simulink model "LinearIntegralAntiWindup"  (R2024b)
settings: Solver=FixedStepAuto  StartTime=0  StopTime=120  FixedStep=0.002  RelTol=1e-3
model workspace (MAT data in the model file):
  Disturbance : Simulink.Parameter (value not decoded)
  ToDrvDesigner : Simulink.Parameter (value not decoded)
values from neighbouring files (symbols this model uses):
  C_af = 80000.0    [VehicleData.sldd]
  C_ar = 80000.0    [VehicleData.sldd]
  g = 9.81    [VehicleData.sldd]
  Iz = 2873.0    [VehicleData.sldd]
  lf = 1.1    [VehicleData.sldd]
  lr = 1.58    [VehicleData.sldd]
  m = 2238.932    [VehicleData.sldd]
symbols that are objects in the model workspace (value not decoded): Disturbance
undefined symbols (not defined in the file or in its folder): phi
libraries: slpidlib x9, SignalEditorBlockLib x1
(part 2 of 3)

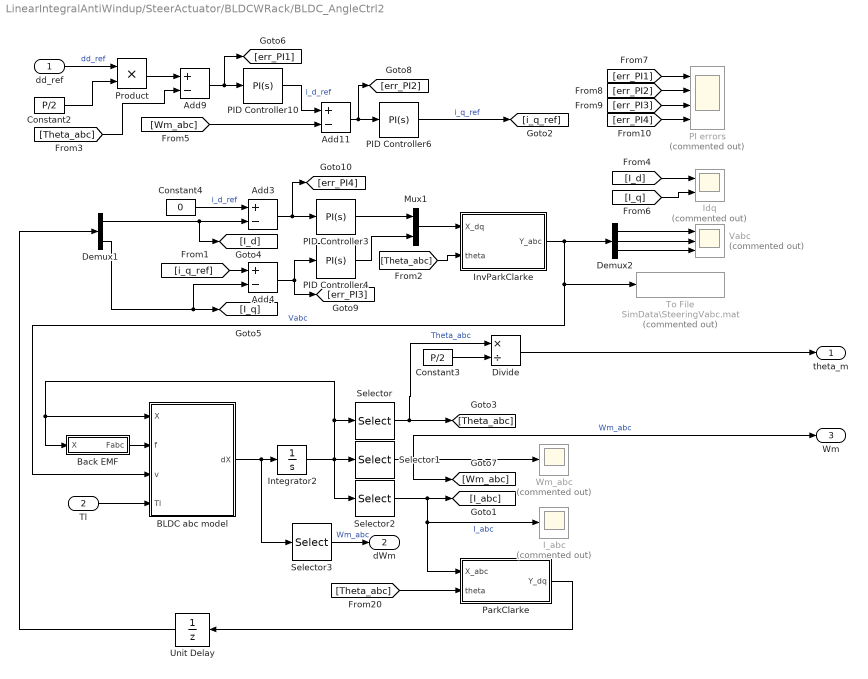
== system LinearIntegralAntiWindup/SteerActuator/BLDCWRack/BLDC_AngleCtrl2 ==
  dd_ref : Inport
  Tl : Inport  Port=2
  Add{3..4,9,11} (4 alike) : Sum  Inputs=+-
  BLDC abc model : MATLAB Function  TreatAsAtomicUnit=on
  Back EMF : MATLAB Function  TreatAsAtomicUnit=on
  Constant2 : Constant  Value=P/2
  Constant3 : Constant  Value=P/2
  Constant4 : Constant  Value=0
  Demux1 : Demux  Outputs=2
  Demux2 : Demux  Outputs=3
  Divide : Product  Inputs=*/
  I_abc : Scope  Commented=on
  Idq : Scope  Commented=on  NumInputPorts=2
  Integrator2 : Integrator  InitialCondition=[0;0;0;0.1;0]
  InvParkClarke : MATLAB Function  TreatAsAtomicUnit=on
  Mux1 : Mux  Inputs=2
  PI errors : Scope  Commented=on  NumInputPorts=4
  PID Controller10 : slpidlib/PID Controller  Controller=PI  Form=Parallel  TimeDomain=Continuous-time  UseExternalTs=off  SampleTime=-1  IntegratorMethod=Forward Euler  FilterMethod=Forward Euler  ControllerParametersSource=internal  P=50  I=2  UseKiTs=off  D=0  UseExternalDerivativeSource=off  N=100  UseFilter=on  TunerSelectOption=Transfer Function Based (PID Tuner App)  InitialConditionSource=internal  InitialConditionForIntegrator=0  InitialConditionForFilter=0  DifferentiatorICPrevScaledInput=0  ExternalReset=none  TrackingMode=off  Kt=1  LimitOutput=off  SatLimitsSource=internal  UpperSaturationLimit=500  LowerSaturationLimit=-500  LinearizeAsGain=on  AntiWindupMode=back-calculation  Kb=1  LimitIntegrator=off  UpperIntegratorSaturationLimit=inf  LowerIntegratorSaturationLimit=-inf  POutMin=[]  POutMax=[]  IOutMin=[]  IOutMax=[]  DOutMin=[]  DOutMax=[]  NOutMin=[]  NOutMax=[]  SumOutMin=[]  SumOutMax=[]  SaturationOutMin=[]  SaturationOutMax=[]  PParamMin=[]  PParamMax=[]  IParamMin=[]  IParamMax=[]  DParamMin=[]  DParamMax=[]  NParamMin=[]  NParamMax=[]  KbParamMin=[]  KbParamMax=[]  KtParamMin=[]  KtParamMax=[]  KbOutMin=[]  KbOutMax=[]  KtOutMin=[]  KtOutMax=[]  IntegratorOutMin=[]  IntegratorOutMax=[]  FilterOutMin=[]  FilterOutMax=[]  SumI1OutMin=[]  SumI1OutMax=[]  SumI2OutMin=[]  SumI2OutMax=[]  SumI3OutMin=[]  SumI3OutMax=[]  SumI4OutMin=[]  SumI4OutMax=[]  SumDOutMin=[]  SumDOutMax=[]  DifferentiatorOutMin=[]  DifferentiatorOutMax=[]  FilterDiffOutCoefMin=[]  FilterDiffOutCoefMax=[]  ReciprocalOutMin=[]  ReciprocalOutMax=[]  SumDenOutMin=[]  SumDenOutMax=[]  SumNumOutMin=[]  SumNumOutMax=[]  DivideOutMin=[]  DivideOutMax=[]  UdiffTsProdOutMin=[]  UdiffTsProdOutMax=[]  NTsProdOutMin=[]  NTsProdOutMax=[]  UintegralTsProdOutMin=[]  UintegralTsProdOutMax=[]  UngainTsProdOutMin=[]  UngainTsProdOutMax=[]  ClampingZeroOutDataTypeStr=Inherit: Inherit via back propagation  ClampingZeroOutMin=[]  ClampingZeroOutMax=[]  FilterDenConstantOutDataTypeStr=Inherit: Inherit via back propagation  FilterDenConstantOutMin=[]  FilterDenConstantOutMax=[]  PCopyOutDataTypeStr=Inherit: Inherit via back propagation  PCopyOutMin=[]  PCopyOutMax=[]  NCopyOutDataTypeStr=Inherit: Inherit via back propagation  NCopyOutMin=[]  NCopyOutMax=[]  IntegratorContinuousStateAttributes=''  IntegratorStateMustResolveToSignalObject=off  IntegratorRTWStateStorageClass=Auto  FilterContinuousStateAttributes=''  FilterStateMustResolveToSignalObject=off  FilterRTWStateStorageClass=Auto  ParallelPVariant=InternalParameters  IdealPVariant=Disabled  IVariant=InternalParameters  DVariant=Disabled  IntegratorVariant=Continuous  SatVariant=Disabled  AWVariant=Passthrough  PCopyVariant=Disabled  TRVariant=Disabled  FdbkBlocksVariant=Forward  IdealPFdbkVariant=Disabled  SatFdbkVariant=Disabled  DerivativeFilterVariant=Disabled  NVariant=Disabled  NCopyVariant=Disabled_SignalSpec  FilterICVariant=Disabled  IntegratorICVariant=InternalICs  ExternalResetVariant=Disabled  TRSumVariant=Passthrough  SumFdbkVariant=Disabled  SumVariant=Sum_PI  TsampFilterVariant=InternalTs  TsampNgainVariant=Passthrough  TsampIntegralVariant=Disabled_SignalSpec  ExternalSaturationOutDataTypeStr=Inherit: Same as second input  DerivativeSourceVariant=Disabled  PreIntVariant=InternalPreInt
  PID Controller3 : slpidlib/PID Controller  Controller=PI  Form=Parallel  TimeDomain=Continuous-time  UseExternalTs=off  SampleTime=-1  IntegratorMethod=Forward Euler  FilterMethod=Forward Euler  ControllerParametersSource=internal  P=30  I=0  UseKiTs=off  D=0  UseExternalDerivativeSource=off  N=100  UseFilter=on  TunerSelectOption=Transfer Function Based (PID Tuner App)  InitialConditionSource=internal  InitialConditionForIntegrator=0  InitialConditionForFilter=0  DifferentiatorICPrevScaledInput=0  ExternalReset=none  TrackingMode=off  Kt=1  LimitOutput=on  SatLimitsSource=internal  UpperSaturationLimit=sqrt(2/3)*13.5  LowerSaturationLimit=-sqrt(2/3)*13.5  LinearizeAsGain=on  AntiWindupMode=back-calculation  Kb=1  LimitIntegrator=off  UpperIntegratorSaturationLimit=inf  LowerIntegratorSaturationLimit=-inf  POutMin=[]  POutMax=[]  IOutMin=[]  IOutMax=[]  DOutMin=[]  DOutMax=[]  NOutMin=[]  NOutMax=[]  SumOutMin=[]  SumOutMax=[]  SaturationOutMin=[]  SaturationOutMax=[]  PParamMin=[]  PParamMax=[]  IParamMin=[]  IParamMax=[]  DParamMin=[]  DParamMax=[]  NParamMin=[]  NParamMax=[]  KbParamMin=[]  KbParamMax=[]  KtParamMin=[]  KtParamMax=[]  KbOutMin=[]  KbOutMax=[]  KtOutMin=[]  KtOutMax=[]  IntegratorOutMin=[]  IntegratorOutMax=[]  FilterOutMin=[]  FilterOutMax=[]  SumI1OutMin=[]  SumI1OutMax=[]  SumI2OutMin=[]  SumI2OutMax=[]  SumI3OutMin=[]  SumI3OutMax=[]  SumI4OutMin=[]  SumI4OutMax=[]  SumDOutMin=[]  SumDOutMax=[]  DifferentiatorOutMin=[]  DifferentiatorOutMax=[]  FilterDiffOutCoefMin=[]  FilterDiffOutCoefMax=[]  ReciprocalOutMin=[]  ReciprocalOutMax=[]  SumDenOutMin=[]  SumDenOutMax=[]  SumNumOutMin=[]  SumNumOutMax=[]  DivideOutMin=[]  DivideOutMax=[]  UdiffTsProdOutMin=[]  UdiffTsProdOutMax=[]  NTsProdOutMin=[]  NTsProdOutMax=[]  UintegralTsProdOutMin=[]  UintegralTsProdOutMax=[]  UngainTsProdOutMin=[]  UngainTsProdOutMax=[]  ClampingZeroOutDataTypeStr=Inherit: Inherit via back propagation  ClampingZeroOutMin=[]  ClampingZeroOutMax=[]  FilterDenConstantOutDataTypeStr=Inherit: Inherit via back propagation  FilterDenConstantOutMin=[]  FilterDenConstantOutMax=[]  PCopyOutDataTypeStr=Inherit: Inherit via back propagation  PCopyOutMin=[]  PCopyOutMax=[]  NCopyOutDataTypeStr=Inherit: Inherit via back propagation  NCopyOutMin=[]  NCopyOutMax=[]  IntegratorContinuousStateAttributes=''  IntegratorStateMustResolveToSignalObject=off  IntegratorRTWStateStorageClass=Auto  FilterContinuousStateAttributes=''  FilterStateMustResolveToSignalObject=off  FilterRTWStateStorageClass=Auto  ParallelPVariant=InternalParameters  IdealPVariant=Disabled  IVariant=InternalParameters  DVariant=Disabled  IntegratorVariant=Continuous  SatVariant=Enabled  AWVariant=BackCalculation  PCopyVariant=Disabled  TRVariant=Disabled  FdbkBlocksVariant=Forward  IdealPFdbkVariant=Disabled  SatFdbkVariant=Disabled  DerivativeFilterVariant=Disabled  NVariant=Disabled  NCopyVariant=Disabled_SignalSpec  FilterICVariant=Disabled  IntegratorICVariant=InternalICs  ExternalResetVariant=Disabled  TRSumVariant=Passthrough  SumFdbkVariant=Disabled  SumVariant=Sum_PI  TsampFilterVariant=InternalTs  TsampNgainVariant=Passthrough  TsampIntegralVariant=Disabled_SignalSpec  ExternalSaturationOutDataTypeStr=Inherit: Same as second input  DerivativeSourceVariant=Disabled  PreIntVariant=InternalPreInt
  PID Controller4 : slpidlib/PID Controller  Controller=PI  Form=Parallel  TimeDomain=Continuous-time  UseExternalTs=off  SampleTime=-1  IntegratorMethod=Forward Euler  FilterMethod=Forward Euler  ControllerParametersSource=internal  P=40  I=80  UseKiTs=off  D=0  UseExternalDerivativeSource=off  N=100  UseFilter=on  TunerSelectOption=Transfer Function Based (PID Tuner App)  InitialConditionSource=internal  InitialConditionForIntegrator=0  InitialConditionForFilter=0  DifferentiatorICPrevScaledInput=0  ExternalReset=none  TrackingMode=off  Kt=1  LimitOutput=on  SatLimitsSource=internal  UpperSaturationLimit=sqrt(2/3)*13.5  LowerSaturationLimit=-sqrt(2/3)*13.5  LinearizeAsGain=on  AntiWindupMode=back-calculation  Kb=1  LimitIntegrator=off  UpperIntegratorSaturationLimit=inf  LowerIntegratorSaturationLimit=-inf  POutMin=[]  POutMax=[]  IOutMin=[]  IOutMax=[]  DOutMin=[]  DOutMax=[]  NOutMin=[]  NOutMax=[]  SumOutMin=[]  SumOutMax=[]  SaturationOutMin=[]  SaturationOutMax=[]  PParamMin=[]  PParamMax=[]  IParamMin=[]  IParamMax=[]  DParamMin=[]  DParamMax=[]  NParamMin=[]  NParamMax=[]  KbParamMin=[]  KbParamMax=[]  KtParamMin=[]  KtParamMax=[]  KbOutMin=[]  KbOutMax=[]  KtOutMin=[]  KtOutMax=[]  IntegratorOutMin=[]  IntegratorOutMax=[]  FilterOutMin=[]  FilterOutMax=[]  SumI1OutMin=[]  SumI1OutMax=[]  SumI2OutMin=[]  SumI2OutMax=[]  SumI3OutMin=[]  SumI3OutMax=[]  SumI4OutMin=[]  SumI4OutMax=[]  SumDOutMin=[]  SumDOutMax=[]  DifferentiatorOutMin=[]  DifferentiatorOutMax=[]  FilterDiffOutCoefMin=[]  FilterDiffOutCoefMax=[]  ReciprocalOutMin=[]  ReciprocalOutMax=[]  SumDenOutMin=[]  SumDenOutMax=[]  SumNumOutMin=[]  SumNumOutMax=[]  DivideOutMin=[]  DivideOutMax=[]  UdiffTsProdOutMin=[]  UdiffTsProdOutMax=[]  NTsProdOutMin=[]  NTsProdOutMax=[]  UintegralTsProdOutMin=[]  UintegralTsProdOutMax=[]  UngainTsProdOutMin=[]  UngainTsProdOutMax=[]  ClampingZeroOutDataTypeStr=Inherit: Inherit via back propagation  ClampingZeroOutMin=[]  ClampingZeroOutMax=[]  FilterDenConstantOutDataTypeStr=Inherit: Inherit via back propagation  FilterDenConstantOutMin=[]  FilterDenConstantOutMax=[]  PCopyOutDataTypeStr=Inherit: Inherit via back propagation  PCopyOutMin=[]  PCopyOutMax=[]  NCopyOutDataTypeStr=Inherit: Inherit via back propagation  NCopyOutMin=[]  NCopyOutMax=[]  IntegratorContinuousStateAttributes=''  IntegratorStateMustResolveToSignalObject=off  IntegratorRTWStateStorageClass=Auto  FilterContinuousStateAttributes=''  FilterStateMustResolveToSignalObject=off  FilterRTWStateStorageClass=Auto  ParallelPVariant=InternalParameters  IdealPVariant=Disabled  IVariant=InternalParameters  DVariant=Disabled  IntegratorVariant=Continuous  SatVariant=Enabled  AWVariant=BackCalculation  PCopyVariant=Disabled  TRVariant=Disabled  FdbkBlocksVariant=Forward  IdealPFdbkVariant=Disabled  SatFdbkVariant=Disabled  DerivativeFilterVariant=Disabled  NVariant=Disabled  NCopyVariant=Disabled_SignalSpec  FilterICVariant=Disabled  IntegratorICVariant=InternalICs  ExternalResetVariant=Disabled  TRSumVariant=Passthrough  SumFdbkVariant=Disabled  SumVariant=Sum_PI  TsampFilterVariant=InternalTs  TsampNgainVariant=Passthrough  TsampIntegralVariant=Disabled_SignalSpec  ExternalSaturationOutDataTypeStr=Inherit: Same as second input  DerivativeSourceVariant=Disabled  PreIntVariant=InternalPreInt
  PID Controller6 : slpidlib/PID Controller  Controller=PI  Form=Parallel  TimeDomain=Continuous-time  UseExternalTs=off  SampleTime=-1  IntegratorMethod=Forward Euler  FilterMethod=Forward Euler  ControllerParametersSource=internal  P=-15  I=-75  UseKiTs=off  D=0  UseExternalDerivativeSource=off  N=100  UseFilter=on  TunerSelectOption=Transfer Function Based (PID Tuner App)  InitialConditionSource=internal  InitialConditionForIntegrator=0  InitialConditionForFilter=0  DifferentiatorICPrevScaledInput=0  ExternalReset=none  TrackingMode=off  Kt=1  LimitOutput=off  SatLimitsSource=internal  UpperSaturationLimit=500  LowerSaturationLimit=-500  LinearizeAsGain=on  AntiWindupMode=back-calculation  Kb=1  LimitIntegrator=off  UpperIntegratorSaturationLimit=inf  LowerIntegratorSaturationLimit=-inf  POutMin=[]  POutMax=[]  IOutMin=[]  IOutMax=[]  DOutMin=[]  DOutMax=[]  NOutMin=[]  NOutMax=[]  SumOutMin=[]  SumOutMax=[]  SaturationOutMin=[]  SaturationOutMax=[]  PParamMin=[]  PParamMax=[]  IParamMin=[]  IParamMax=[]  DParamMin=[]  DParamMax=[]  NParamMin=[]  NParamMax=[]  KbParamMin=[]  KbParamMax=[]  KtParamMin=[]  KtParamMax=[]  KbOutMin=[]  KbOutMax=[]  KtOutMin=[]  KtOutMax=[]  IntegratorOutMin=[]  IntegratorOutMax=[]  FilterOutMin=[]  FilterOutMax=[]  SumI1OutMin=[]  SumI1OutMax=[]  SumI2OutMin=[]  SumI2OutMax=[]  SumI3OutMin=[]  SumI3OutMax=[]  SumI4OutMin=[]  SumI4OutMax=[]  SumDOutMin=[]  SumDOutMax=[]  DifferentiatorOutMin=[]  DifferentiatorOutMax=[]  FilterDiffOutCoefMin=[]  FilterDiffOutCoefMax=[]  ReciprocalOutMin=[]  ReciprocalOutMax=[]  SumDenOutMin=[]  SumDenOutMax=[]  SumNumOutMin=[]  SumNumOutMax=[]  DivideOutMin=[]  DivideOutMax=[]  UdiffTsProdOutMin=[]  UdiffTsProdOutMax=[]  NTsProdOutMin=[]  NTsProdOutMax=[]  UintegralTsProdOutMin=[]  UintegralTsProdOutMax=[]  UngainTsProdOutMin=[]  UngainTsProdOutMax=[]  ClampingZeroOutDataTypeStr=Inherit: Inherit via back propagation  ClampingZeroOutMin=[]  ClampingZeroOutMax=[]  FilterDenConstantOutDataTypeStr=Inherit: Inherit via back propagation  FilterDenConstantOutMin=[]  FilterDenConstantOutMax=[]  PCopyOutDataTypeStr=Inherit: Inherit via back propagation  PCopyOutMin=[]  PCopyOutMax=[]  NCopyOutDataTypeStr=Inherit: Inherit via back propagation  NCopyOutMin=[]  NCopyOutMax=[]  IntegratorContinuousStateAttributes=''  IntegratorStateMustResolveToSignalObject=off  IntegratorRTWStateStorageClass=Auto  FilterContinuousStateAttributes=''  FilterStateMustResolveToSignalObject=off  FilterRTWStateStorageClass=Auto  ParallelPVariant=InternalParameters  IdealPVariant=Disabled  IVariant=InternalParameters  DVariant=Disabled  IntegratorVariant=Continuous  SatVariant=Disabled  AWVariant=Passthrough  PCopyVariant=Disabled  TRVariant=Disabled  FdbkBlocksVariant=Forward  IdealPFdbkVariant=Disabled  SatFdbkVariant=Disabled  DerivativeFilterVariant=Disabled  NVariant=Disabled  NCopyVariant=Disabled_SignalSpec  FilterICVariant=Disabled  IntegratorICVariant=InternalICs  ExternalResetVariant=Disabled  TRSumVariant=Passthrough  SumFdbkVariant=Disabled  SumVariant=Sum_PI  TsampFilterVariant=InternalTs  TsampNgainVariant=Passthrough  TsampIntegralVariant=Disabled_SignalSpec  ExternalSaturationOutDataTypeStr=Inherit: Same as second input  DerivativeSourceVariant=Disabled  PreIntVariant=InternalPreInt
  ParkClarke : MATLAB Function  TreatAsAtomicUnit=on
  Product : Product
  Selector : Selector  InputPortWidth=5  IndexOptions=Index vector (dialog)  Indices=[5]  OutputSizes=1
  Selector1 : Selector  InputPortWidth=5  IndexOptions=Index vector (dialog)  Indices=[4]  OutputSizes=1
  Selector2 : Selector  InputPortWidth=5  IndexOptions=Index vector (dialog)  Indices=[1:3]  OutputSizes=1
  Selector3 : Selector  InputPortWidth=5  IndexOptions=Index vector (dialog)  Indices=[4]  OutputSizes=1
  To File : ToFile  Commented=on  Filename=SimData\SteeringVabc.mat  SaveFormat=Timeseries
  Unit Delay : UnitDelay  InitialCondition=[0;0]  SampleTime=-1  HasFrameUpgradeWarning=on
  Vabc : Scope  Commented=on  NumInputPorts=3
  Wm_abc : Scope  Commented=on
  theta_m : Outport
  dWm : Outport  Port=2
  Wm : Outport  Port=3
  wires:
  Constant4/1 -> Add3/1  "i_d_ref"
  Back EMF/1(Fabc) -> BLDC abc model/2(f)
  Unit Delay/1 -> Demux1/1
  Add11/1 -> PID Controller6/1, [err_PI2]
  Add9/1 -> [err_PI1], PID Controller10/1
  Demux1/2 -> [I_q], Add4/2
  [Wm_abc] -> Add11/2
  [Theta_abc] -> Add9/2
  Selector2/1 -> ParkClarke/1(X_abc), I_abc/1, [I_abc]  "I_abc"
  Mux1/1 -> InvParkClarke/1(X_dq)
  [Theta_abc] -> ParkClarke/2(theta)
  [Theta_abc] -> InvParkClarke/2(theta)
  Selector/1 -> [Theta_abc], Divide/1  "Theta_abc"
  PID Controller3/1 -> Mux1/1
  ParkClarke/1(Y_dq) -> Unit Delay/1
  Tl/1 -> BLDC abc model/4(Tl)
  InvParkClarke/1(Y_abc) -> BLDC abc model/3(v), To File/1, Demux2/1  "Vabc"
  PID Controller4/1 -> Mux1/2
  BLDC abc model/1(dX) -> Selector3/1, Integrator2/1
  Selector1/1 -> Wm/1, [Wm_abc], Wm_abc/1  "Wm_abc"
  Add4/1 -> [err_PI3], PID Controller4/1
  Demux1/1 -> [I_d], Add3/2
  Add3/1 -> PID Controller3/1, [err_PI4]
  Integrator2/1 -> BLDC abc model/1(X), Back EMF/1(X), Selector/1, Selector2/1, Selector1/1
  [i_q_ref] -> Add4/1
  Product/1 -> Add9/1
  dd_ref/1 -> Product/1  "dd_ref"
  Constant2/1 -> Product/2
  Divide/1 -> theta_m/1
  Constant3/1 -> Divide/2
  [err_PI1] -> PI errors/1
  [err_PI2] -> PI errors/2
  [err_PI3] -> PI errors/3
  [err_PI4] -> PI errors/4
  Demux2/1 -> Vabc/1
  Demux2/2 -> Vabc/2
  Demux2/3 -> Vabc/3
  PID Controller6/1 -> [i_q_ref]  "i_q_ref"
  PID Controller10/1 -> Add11/1  "i_d_ref"
  Selector3/1 -> dWm/1  "Wm_abc"
  [I_d] -> Idq/1
  [I_q] -> Idq/2

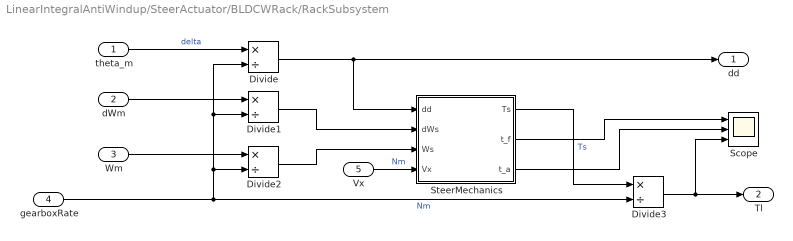
== system LinearIntegralAntiWindup/SteerActuator/BLDCWRack/RackSubsystem ==
  theta_m : Inport
  dWm : Inport  Port=2
  Wm : Inport  Port=3
  gearboxRate : Inport  Port=4
  Vx : Inport  Port=5
  Divide{,1..3} (4 alike) : Product  Inputs=*/
  Scope : Scope  NumInputPorts=3
  SteerMechanics : MATLAB Function  TreatAsAtomicUnit=on
  dd : Outport
  Tl : Outport  Port=2
  wires:
  theta_m/1 -> Divide/1  "delta"
  gearboxRate/1 -> Divide2/2, Divide1/2, Divide/2, Divide3/2  "Nm"
  dWm/1 -> Divide1/1
  Wm/1 -> Divide2/1
  Divide/1 -> dd/1, SteerMechanics/1(dd)
  Divide1/1 -> SteerMechanics/2(dWs)
  Divide2/1 -> SteerMechanics/3(Ws)
  SteerMechanics/1(Ts) -> Divide3/1  "Ts"
  Divide3/1 -> Scope/3, Tl/1
  SteerMechanics/2(t_f) -> Scope/1
  SteerMechanics/3(t_a) -> Scope/2
  Vx/1 -> SteerMechanics/4(Vx)  "Nm"

== matlab function LinearIntegralAntiWindup/LateralController/HOSMC_IntegralBlocksSuperTwisting/MATLAB Function3 ==
  data: u input; y output
function y = fcn(u)
L = pi/8;
e = 1;

y = L.*tanh(u./e);

== matlab function LinearIntegralAntiWindup/LateralController/DirectLyapunov ==
  data: U output size=1; E input; Vx input; dPsi_des input; C_af parameter; g parameter; C_ar parameter; lf parameter; lr parameter; Iz parameter; m parameter
% ******************* Lateral dynamic controller *********************
%*********************************************************************
% Author: L.Arturo Torres-Romero
% Date: 22-10-2020
% This controller controlls the direction of a car, based in the dynamics
% described  in the next link and using the Direct Lyapunov formulation: 
% https://www.researchgate.net/publication/340166902_LATERAL_VEHICLE_DYNAMICS_AND_CONTROLLERS_DESIGN
%
%ALCALÁ, Eugenio, et al. Comparison of two non-linear model-based control strategies for autonomous vehicles. 
% En 2016 24th Mediterranean Conference on Control and Automation (MED). IEEE, 2016. p. 846-851.
%******************* PARAMETERS DESCRIPTIONS **********************
%******************************************************************
% m: vehicle mass
% g: gravity
% C_af : Cornering  stiffness  of  front  wheels.
% C_ar : Cornering  stiffness  of  rear  wheels.
% lf : distance fron the center of gravity to the front wheel axis.
% lr : distance fron the center of gravity to the rear wheel axis.
% Iz : this is the momentum of inertia of the vehicle respect the z axis.
%******************************************************************
%******************* INPUTS DESCRIPTIONS **************************
%******************************************************************
% E:   (column vector)[e1;de1;e2;de2] states of the state space of 
%       the system that includes the errors as follows:
%      e1  : is the lateral position error respect the road.
%      de1 : derivative of e1.
%      e2  : is the yaw angle error with respect the road. 
%      de2 : derivarive of the e2.
% Vx: Logitudinal velocity.

%******************************************************************
% ******************* OUTPUTS DESCRIPTIONS ************************
%******************************************************************
% U: control coutput in radians. Angle of the frontal wheels respect to the
%    longitudinal axis
% isCtrl: when true means that the matrix Mc has full rank, and hence, the
%         system is controllable
%******************************************************************

function U = DirectLyapunovCtrl(E, Vx,dPsi_des, C_af, g, C_ar, lf, lr, Iz, m) % pd polos deseados

psi_e = E(3);
y_e = E(1);
L = lf+lr;
k2 = 1.1;
k3 = 3;

dPsi_ctrl = dPsi_des -k2*Vx*(sin(psi_e)/psi_e)*y_e - k3*psi_e;

ctrlVal = atan((L*dPsi_ctrl)/Vx);


U = real(ctrlVal);

== matlab function LinearIntegralAntiWindup/LateralController/HOSMC_IntegralNestedST/MATLAB Function1 ==
  data: u input; y output
function y = fcn(u)
L = pi/32;
e = 1;

y = L.*tanh(u./e);

== matlab function LinearIntegralAntiWindup/LateralController/SMC_Alcala/AlcalaSMC ==
  data: U output size=1; E input; Vx input; dPsi_des input; dx_e input; ddPsi_des input; C_af parameter; g parameter; C_ar parameter; lf parameter; lr parameter; Iz parameter; m parameter
% ******************* Lateral dynamic controller *********************
%*********************************************************************
% Author: L.Arturo Torres-Romero
% Date: 22-10-2020
% This controller controlls the direction of a car, based in the dynamics
% described  in the next link and using the Direct Lyapunov formulation: 
% https://www.researchgate.net/publication/340166902_LATERAL_VEHICLE_DYNAMICS_AND_CONTROLLERS_DESIGN
%
%ALCALÁ, Eugenio, et al. Comparison of two non-linear model-based control strategies for autonomous vehicles. 
% En 2016 24th Mediterranean Conference on Control and Automation (MED). IEEE, 2016. p. 846-851.
%******************* PARAMETERS DESCRIPTIONS **********************
%******************************************************************
% m: vehicle mass
% g: gravity
% C_af : Cornering  stiffness  of  front  wheels.
% C_ar : Cornering  stiffness  of  rear  wheels.
% lf : distance fron the center of gravity to the front wheel axis.
% lr : distance fron the center of gravity to the rear wheel axis.
% Iz : this is the momentum of inertia of the vehicle respect the z axis.
%******************************************************************
%******************* INPUTS DESCRIPTIONS **************************
%******************************************************************
% E:   (column vector)[e1;de1;e2;de2] states of the state space of 
%       the system that includes the errors as follows:
%      e1  : is the lateral position error respect the road.
%      de1 : derivative of e1.
%      e2  : is the yaw angle error with respect the road. 
%      de2 : derivarive of the e2.
% Vx: Logitudinal velocity.

%******************************************************************
% ******************* OUTPUTS DESCRIPTIONS ************************
%******************************************************************
% U: control coutput in radians. Angle of the frontal wheels respect to the
%    longitudinal axis
% isCtrl: when true means that the matrix Mc has full rank, and hence, the
%         system is controllable
%******************************************************************

function U = SMC_Ctrl_1(E, Vx,dPsi_des,dx_e,ddPsi_des, C_af, g, C_ar, lf, lr, Iz, m) % pd polos deseados
y_e = E(1);
dy_e = E(2);
psi_e = E(3);
dpsi_e = E(4);
x_e = E(5);


L = lf+lr;
k2 = 2;
k3 = 2.55;
P2 = 3.7;
Q2 = 0.3;

s2 = dy_e +k2*y_e + k3*psi_e;

dPsi_ctrl = dPsi_des + (-P2*s2 -Q2*sign(s2) -k2*dy_e + ddPsi_des*x_e + dPsi_des*dx_e  -Vx*sin(psi_e))/(Vx*sin(psi_e)+k3);

ctrlVal = atan((L*dPsi_ctrl)/Vx);

U = real(ctrlVal);

== matlab function LinearIntegralAntiWindup/LateralController/SMC_UrbanoPathFollowing/SMC_UrbanoPathFollowing ==
  data: U output size=1; E input; Vx input; dPsi_des input; d_d input; C_af parameter; g parameter; C_ar parameter; lf parameter; lr parameter; Iz parameter; m parameter; dd_d output
% ******************* Lateral dynamic controller *********************
%*********************************************************************
% Author: L.Arturo Torres-Romero
% Date: 22-10-2023
% This controller controlls the direction of a car, based on the path
% following controller described  in the next paper and link: 
%
%SOLEA, Razvan; NUNES, Urbano. Trajectory planning and sliding-mode control based trajectory-tracking for cybercars. 
% Integrated Computer-Aided Engineering, 2007, vol. 14, no 1, p. 33-47.
%
%https://www.researchgate.net/publication/228634486_Trajectory_planning_and_sliding-mode_control_based_trajectory-tracking_for_cybercars
%SOLEA, Razvan; NUNES, Urbano. Trajectory planning and sliding-mode control based trajectory-tracking for cybercars.
%Integrated Computer-Aided Engineering, 2007, vol. 14, no 1, p. 33-47.
%
%******************* PARAMETERS DESCRIPTIONS **********************
%******************************************************************
% m: vehicle mass
% g: gravity
% C_af : Cornering  stiffness  of  front  wheels.
% C_ar : Cornering  stiffness  of  rear  wheels.
% lf : distance fron the center of gravity to the front wheel axis.
% lr : distance fron the center of gravity to the rear wheel axis.
% Iz : this is the momentum of inertia of the vehicle respect the z axis.
%******************************************************************
%******************* INPUTS DESCRIPTIONS **************************
%******************************************************************
% E:   (column vector)[e1;de1;e2;de2] states of the state space of 
%       the system that includes the errors as follows:
%      e1  : is the lateral position error respect the road.
%      de1 : derivative of e1.
%      e2  : is the yaw angle error with respect the road. 
%      de2 : derivarive of the e2.
% Vx: Logitudinal velocity.

%******************************************************************
% ******************* OUTPUTS DESCRIPTIONS ************************
%******************************************************************
% U: control coutput in radians. Angle of the frontal wheels respect to the
%    longitudinal axis
%******************************************************************

function [U, dd_d] = SMC_Ctrl_1(E, Vx,dPsi_des, d_d, C_af, g, C_ar, lf, lr, Iz, m) % pd polos deseados
y_e = E(1);
dy_e = E(2);
psi_e = E(3);
dpsi_e = E(4);

L = lf+lr;
k = 0.5;
k0 = 0.05;
q1 = 1;
q2 = 1;
p1 = 1;
p2 = 1;
Lh = 6.5; % this lenght was obtained based in the 5 points ahead of the C.G. for refference aprx. See GetRefference block

s = dy_e + k*y_e + k0*sign(y_e)*psi_e;

if Lh == 0   % Look-ahead = 0. TODO
    ctrlVal = 0;


else   % Look-ahead <> 0|
    Q = q1;
    P = p1;
    tmp1 = (L*(cos(d_d))^2)/(Vx*Lh*cos(dpsi_e)^2);
    tmp2 = -Q*s -P*sign(s)-k*dy_e -Vx*dpsi_e*cos(psi_e) + Lh*dpsi_e^2*sin(psi_e) - k0*sign(y_e)*dpsi_e;
    dd_d = tmp1*tmp2;
    ctrlVal = real(d_d); 
end

U = real(ctrlVal);

== matlab function LinearIntegralAntiWindup/LateralController/AckermanCtrl ==
  data: U output size=1; E input; Vx input; C_af parameter; g parameter; C_ar parameter; lf parameter; lr parameter; Iz parameter; m parameter
% ******************* Lateral dynamic controller *********************
%*********************************************************************
% Author: L.Arturo Torres-Romero
% Date: 22-10-2020
% This controller controlls the direction of a car, based in the dynamics
% described  in the next link and using the Ackerman formulation: 
% https://www.researchgate.net/publication/340166902_LATERAL_VEHICLE_DYNAMICS_AND_CONTROLLERS_DESIGN
%******************* PARAMETERS DESCRIPTIONS **********************
%******************************************************************
% m: vehicle mass
% g: gravity
% C_af : Cornering  stiffness  of  front  wheels.
% C_ar : Cornering  stiffness  of  rear  wheels.
% lf : distance fron the center of gravity to the front wheel axis.
% lr : distance fron the center of gravity to the rear wheel axis.
% Iz : this is the momentum of inertia of the vehicle respect the z axis.
%******************************************************************
%******************* INPUTS DESCRIPTIONS **************************
%******************************************************************
% E:   (column vector)[e1;de1;e2;de2] states of the state space of 
%       the system that includes the errors as follows:
%      e1  : is the lateral position error respect the road.
%      de1 : derivative of e1.
%      e2  : is the yaw angle error with respect the road. 
%      de2 : derivarive of the e2.
% Vx: Logitudinal velocity.

%******************************************************************
% ******************* OUTPUTS DESCRIPTIONS ************************
%******************************************************************
% U: control coutput in radians. Angle of the frontal wheels respect to the
%    longitudinal axis
% isCtrl: when true means that the matrix Mc has full rank, and hence, the
%         system is controllable
%******************************************************************

function U = AckermanLateralCtrl(E, Vx, C_af, g, C_ar, lf, lr, Iz, m) % pd polos deseados
X = [0; 0; 0; 0];
X(1) = E(1);
X(2) = E(2);
X(3) = E(3);
X(4) = E(4);
%**************************************************
%******* Matrix A formulation *********************
A22 = -(2*C_af + 2*C_ar)/(m*Vx);
A23 = (2*C_af + 2*C_ar)/m;
A24 = (-2*C_af*lf + 2*C_ar*lr)/(m*Vx);
A42 = -(2*C_af*lf - 2*C_ar*lr)/(Iz*Vx);
A43 = (2*C_af*lf - 2*C_ar*lr)/Iz;
A44 = -(2*C_af*lf^2 + 2*C_ar*lr^2)/(Iz*Vx);

A = [0 1 0 0;0 A22 A23 A24;0 0 0 1;0 A42 A43 A44];
%**************************************************

%**************************************************
%******* Matrix B1 formulation ********************
B1_2 = 2*C_af/m;
B1_4 = 2*C_af*lf/Iz;

B1 = [0;B1_2;0;B1_4];
%***************************************************

%***************************************************
%******* Matrix B2 formulation *********************
B2_2 = -(2*C_af*lf - 2*C_ar*lr)/(m*Vx) - Vx;
B2_4 = -(2*C_af*lf^2 + 2*C_ar*lr^2)/(Iz*Vx);

B2 = [0;B2_2;0;B2_4];
%***************************************************


%***************************************************
%******* Matrix B3 formulation *********************
B3 = [0;g;0;0];
%***************************************************


%***************************************************
%******* Verification of controllability and output 
% calculation of the controller
%**************************************************
ctrlVal = 0;
Mc = [B1 A*B1 A^2*B1 A^3*B1];
rankVal = rank(Mc);
    if rankVal < size(A,1)
        %disp('Not completely state controllable');
        isCtrl = 0;
        ctrlVal = 0;
    else
        %disp('Completely state controllable');
        isCtrl = 1;
        % Pole placement
        Pd =[-10-3i -8+3i -15 -19]; %[-5-3i -5+3i -7 -10]
        %Pd =[-2 -2 -2 -2];

        H = (A- Pd(1)*eye(4)) * (A- Pd(2)*eye(4)) * (A- Pd(3)*eye(4)) * (A- Pd(4)*eye(4));

        %ackerman formula
        K = [0 0 0 1]*Mc^-1*H;
        ctrlVal = -K*X;  
    end


U = real(ctrlVal);

== matlab function LinearIntegralAntiWindup/LateralController/SMC_Alcala/LevantDiff/Levant ==
  data: dX output; X input; u_ref input; lambda input; alpha input
%*************************************************
% Author: L.Arturo Torres-Romero
% based on 
% Levant A. (1998). Robust exact differentiation via sliding mode technique. 
% Automatica, 34(3), 379-384
%*************************************************

function dX = LevantDiff(X, u_ref, lambda, alpha) 
eta_u0=X(1);    eta_u1= X(2); 

 
%Levant differenciator
 d_eta_u0=eta_u1-lambda*sqrt(abs(eta_u0-u_ref))*sign(eta_u0-u_ref);
 d_eta_u1=-alpha*sign(eta_u0-u_ref);
      
dX = [d_eta_u0;d_eta_u1];
end

== matlab function LinearIntegralAntiWindup/LateralController/SMC_Alcala/LevantDiff1/Levant ==
  data: dX output; X input; u_ref input; lambda input; alpha input
%*************************************************
% Author: L.Arturo Torres-Romero
% based on 
% Levant A. (1998). Robust exact differentiation via sliding mode technique. 
% Automatica, 34(3), 379-384
%*************************************************

function dX = LevantDiff(X, u_ref, lambda, alpha) 
eta_u0=X(1);    eta_u1= X(2); 

 
%Levant differenciator
 d_eta_u0=eta_u1-lambda*sqrt(abs(eta_u0-u_ref))*sign(eta_u0-u_ref);
 d_eta_u1=-alpha*sign(eta_u0-u_ref);
      
dX = [d_eta_u0;d_eta_u1];
end

== matlab function LinearIntegralAntiWindup/SteerActuator/BLDCWRack/BLDC_AngleCtrl2/BLDC abc model ==
  data: X input; f input; v input; dX output; Tl input; R parameter; L parameter; M parameter; J parameter; b parameter; P parameter; lambda parameter
function dX = fcn(X,f,v,Tl, R, L, M, J, b, P, lambda)
% X = [i_a; i_b; i_c; wm; theta_elec]
% f = [f1; f2; f3]  (0..1)
% v = [v1; v2; v3]  (example v = 12.*f)
% Tl = scalar torque load)
% lambda = ke = kt (V·s/rad = N·m/A)
% P = poles qty (pole pairs = P/2
%
% delivers dX = [di_a; di_b; di_c; dwm; dtheta_elec]

% sanity checks
if numel(f)~=3 || numel(v)~=3
    error('f and v must be vectors 3x1.');
end

% effective electric parameters
L_eff = L - M;
if L_eff <= 0
    error('L - M must be possitive. Check M.');
end


% states
i_a = X(1); i_b = X(2); i_c = X(3);
wm  = X(4); theta = X(5);


% electric equations (phase to phase)
di_a = ( v(1) - R*i_a - lambda * f(1) * wm ) / L_eff;
di_b = ( v(2) - R*i_b - lambda * f(2) * wm ) / L_eff;
di_c = ( v(3) - R*i_c - lambda * f(3) * wm ) / L_eff;

% Mechanic equations
T_elec = lambda*( f(1)*i_a + f(2)*i_b + f(3)*i_c ); % torque eléctrico
dwm = ( T_elec - b*wm - Tl ) / J;


% Electric angle
dtheta = (P/2) * wm;

dX = [di_a; di_b; di_c; dwm; dtheta];

end

== matlab function LinearIntegralAntiWindup/MATLAB Function1 ==
  settings: updateMethod=DISCRETE
  data: u input; maxVal output; meanVal output
function [maxVal, meanVal] = statsSignal(u)
%#codegen

% Variables persistentes para acumular datos
persistent max_so_far sum_so_far count_so_far

if isempty(max_so_far)
    max_so_far  = -inf;   % Valor inicial muy bajo
    sum_so_far  = 0;
    count_so_far = 0;
end

% Actualizar máximo
if u > max_so_far
    max_so_far = u;
end

% Acumular para promedio
sum_so_far = sum_so_far + u;
count_so_far = count_so_far + 1;

% Calcular promedio
meanVal = sum_so_far / count_so_far;

% Salida de máximo
maxVal = max_so_far;

== matlab function LinearIntegralAntiWindup/LateralController/SMC_Conventional1 ==
  data: U output size=1; E input; Vx input; C_af parameter; g parameter; C_ar parameter; lf parameter; lr parameter; Iz parameter; m parameter
% ******************* Lateral dynamic controller *********************
%*********************************************************************
% Author: L.Arturo Torres-Romero
% Date: 22-10-2020
% This controller controlls the direction of a car, based in the dynamics
% described  in the next link and using the conventional sliding mode control 
% formulation with the procedure of converting to regular form: 
% https://www.researchgate.net/publication/340166902_LATERAL_VEHICLE_DYNAMICS_AND_CONTROLLERS_DESIGN
%******************* PARAMETERS DESCRIPTIONS **********************
%******************************************************************
% m: vehicle mass
% g: gravity
% C_af : Cornering  stiffness  of  front  wheels.
% C_ar : Cornering  stiffness  of  rear  wheels.
% lf : distance fron the center of gravity to the front wheel axis.
% lr : distance fron the center of gravity to the rear wheel axis.
% Iz : this is the momentum of inertia of the vehicle respect the z axis.
%******************************************************************
%******************* INPUTS DESCRIPTIONS **************************
%******************************************************************
% E:   (column vector)[e1;de1;e2;de2] states of the state space of 
%       the system that includes the errors as follows:
%      e1  : is the lateral position error respect the road.
%      de1 : derivative of e1.
%      e2  : is the yaw angle error with respect the road. 
%      de2 : derivarive of the e2.
% Vx: Logitudinal velocity.

%******************************************************************
% ******************* OUTPUTS DESCRIPTIONS ************************
%******************************************************************
% U: control coutput in radians. Angle of the frontal wheels respect to the
%    longitudinal axis
% isCtrl: when true means that the matrix Mc has full rank, and hence, the
%         system is controllable
%******************************************************************

function U = SMC_ConventionalCtrl(E, Vx, C_af, g, C_ar, lf, lr, Iz, m) % pd polos deseados
X = [0; 0; 0; 0];
X(1) = E(1);
X(2) = E(2);
X(3) = E(3);
X(4) = E(4);
n = 16;
lambda_1 = -1;
lambda_2 = -2;
%**************************************************
%******* Matrix A formulation *********************
A22 = -(2*C_af + 2*C_ar)/(m*Vx);
A23 = (2*C_af + 2*C_ar)/m;
A24 = (-2*C_af*lf + 2*C_ar*lr)/(m*Vx);
A42 = -(2*C_af*lf - 2*C_ar*lr)/(Iz*Vx);
A43 = (2*C_af*lf - 2*C_ar*lr)/Iz;
A44 = -(2*C_af*lf^2 + 2*C_ar*lr^2)/(Iz*Vx);

A = [0 1 0 0;0 A22 A23 A24;0 0 0 1;0 A42 A43 A44];
%**************************************************

%**************************************************
%******* Matrix B1 formulation ********************
B1_2 = 2*C_af/m;
B1_4 = 2*C_af*lf/Iz;

B1 = [0;B1_2;0;B1_4];
%***************************************************

%***************************************************
%******* Matrix B2 formulation *********************
B2_2 = -(2*C_af*lf - 2*C_ar*lr)/(m*Vx) - Vx;
B2_4 = -(2*C_af*lf^2 + 2*C_ar*lr^2)/(Iz*Vx);

B2 = [0;B2_2;0;B2_4];
%***************************************************


%***************************************************
%******* Matrix B3 formulation *********************
B3 = [0;g;0;0];
%***************************************************
x1 = X(1);
x2 = X(2);
x3 = X(3);
x4 = X(4);

%%%%%% this is with S2 = inv(B_2)
% sigma1 = -(lambda_2*x1 - x2 + lambda_2*x3)/B1_2;
% sigma2 = -(lambda_1*x1 - x4 + lambda_1*x3)/B1_4;
% u1 = -(A22*x2 + A23*x3 + A24*x4 - lambda_2*x2 - lambda_2*x4 + B1_2*n*sign(sigma1))/B1_2;
% u2 = -(A42*x2 + A43*x3 + A44*x4 - lambda_1*x2 - lambda_1*x4 + B1_4*n*sign(sigma2))/B1_4;


%%%%%% this is with S2 = eye(2)
sigma1 = -(abs(B1_4)*(lambda_1*x1 - x4 + lambda_1*x3))/B1_4;
sigma2 = -(abs(B1_2)*(lambda_2*x1 - x2 + lambda_2*x3))/B1_2;
u1 = -(A42*x2 + A43*x3 + A44*x4 - lambda_1*x2 - lambda_1*x4 + n*sign(B1_4)*sign(sigma1))/B1_4;
u2 = -(A22*x2 + A23*x3 + A24*x4 - lambda_2*x2 - lambda_2*x4 + n*sign(B1_2)*sign(sigma2))/B1_2;

ctrlVal =  (u2+u1)/2;

U = real(ctrlVal);    



%*****************************************************************************
%******* Live script for help in calculus of the controller ************
% 
% format rational
% syms A B Q R Tr B1_2 B1_4 A22 A23 A24 A42 A43 A44
% A = [0 1 0 0;0 A22 A23 A24;0 0 0 1;0 A42 A43 A44]
% B = [0 0;B1_2 0;0 0;0 B1_4]
% 
% [Q R] = qr(sym(B))
% 
% Tr= flipud(Q') % we need the cero part in the superior part
% rank(Tr)
% 
% B_ = Tr*B
% 
% A_ = Tr*A*inv(Tr)
% 
% % A_ matrix partition
% A_11 = A_(1:2,1:2)
% A_12 = A_(1:2,3:4)
% A_21 = A_(3:4,1:2)
% A_22 = A_(3:4,3:4)
% 
% syms M M11 M12 M21 M22 lambda_1 lambda_2
% M = [M11 M12;M21 M22];
% eqeigen = [lambda_1;lambda_2] == A_11 - A_12*M;
% H = solve(eqeigen,M);
% M_ = [H.M11 H.M12;H.M21 H.M22]
% 
% S2 = eye(2);
% %S2 = inv(B_(3:4,:))
% S = S2*[M_ eye(2)]*Tr;
% disp("surface S: ")
% expand(S)
% 
% syms n sigma_ x1 x2 x3 x4 u1 u2
% X = [x1;x2;x3;x4];
% U = [u1;u2];
% 
% SIGMA = S*X;
% Sigma_1 = simplify(SIGMA(1))
% Sigma_2 = simplify(SIGMA(2))
% 
% eqsolution = -n*sign(sigma_) == S*(A*X + B*U)
% sol1 = solve(eqsolution(1),u2);
% sol2 = solve(eqsolution(2),u1);
% 
% simplify(sol1)
% simplify(sol2)

== matlab function LinearIntegralAntiWindup/SteerActuator/BLDCWRack/BLDC_AngleCtrl2/Back EMF ==
  data: X input; Fabc output
function Fabc = fcn(X)
Fabc = [0;0;0];
    theta = mod(X(5),2*pi); %X(4)
    %theta = mod(X,2*pi);
    
    if (0<=theta)&&(theta<(pi/6))
        Fa = (6/pi)*theta;
    elseif ((pi/6)<=theta)&&(theta<(5*pi/6))
        Fa = 1;
    elseif ((5*pi/6<=theta))&&(theta<(7*pi/6))
        Fa = (6/pi)*(pi-theta);
    elseif ((7*pi/6)<=theta)&&(theta<(11*pi/6))
        Fa = -1;
    elseif ((11*pi/6)<=theta)&&(theta<(2*pi))
        Fa = (6/pi)*(theta-2*pi);
    else
        Fa = NaN;
    end
    
    if (0<=theta)&&(theta<(3*pi/6))
        Fb = -1;
    elseif ((3*pi/6)<=theta)&&(theta<(5*pi/6))
        Fb = (6/pi)*(theta-(2*pi)/3);
    elseif ((5*pi/6)<=theta)&&(theta<(9*pi/6))
        Fb = 1;
    elseif ((9*pi/6)<=theta)&&(theta<(11*pi/6))
        Fb = (6/pi)*(-theta+(5*pi)/3);
    elseif ((11*pi/6)<=theta)&&(theta<(2*pi))
        Fb = -1;
    else
        Fb = NaN;
    end
    
    if (0<=theta)&&(theta<(pi/6))
        Fc = 1;
    elseif ((pi/6)<=theta)&&(theta<(3*pi/6))
        Fc = (6/pi)*(pi/3-theta);
    elseif ((3*pi/6)<=theta)&&(theta<(7*pi/6))
        Fc = -1;
    elseif ((7*pi/6)<=theta)&&(theta<(9*pi/6))
        Fc = (6/pi)*(theta-(4*pi)/3);
    elseif ((9*pi/6)<=theta)&&(theta<(2*pi))
        Fc = 1;
    else
        Fc = NaN; 
    end
    
    
%     
     %Fa = sin(theta);
     %Fb = sin(theta - 2*pi/3);
     %Fc = sin(theta + 2*pi/3);
    
    Fabc = [Fa;Fb;Fc];
end

== matlab function LinearIntegralAntiWindup/SteerActuator/BLDCWRack/BLDC_AngleCtrl2/InvParkClarke ==
  data: X_dq input; Y_abc output; theta input
function Y_abc = fcn(X_dq, theta)
X_dq0 = [0;0;0];
X_dq0 = [X_dq; 0];

%inverse Park-Clarke power invariant
iT_PC = sqrt(2/3)*[cos(theta)          -sin(theta)            1/sqrt(2); ...
                  cos(theta-2*pi/3)   -sin(theta-2*pi/3)     1/sqrt(2); ...
                  cos(theta+2*pi/3)   -sin(theta+2*pi/3)     1/sqrt(2)];
%               
              
 %inverse Park-Clarke amplitude invariant
% iT_PC = [cos(theta)          -sin(theta)            1; ...
%          cos(theta-2*pi/3)   -sin(theta-2*pi/3)     1; ...
%          cos(theta+2*pi/3)   -sin(theta+2*pi/3)     1];



Y_abc =iT_PC*X_dq0;
end

== matlab function LinearIntegralAntiWindup/SteerActuator/BLDCWRack/BLDC_AngleCtrl2/ParkClarke ==
  data: X_abc input; Y_dq output; theta input
function Y_dq = fcn(X_abc, theta)

% Park clarke transform eliminating the third element
PC_T = (sqrt(2)/2)*[sqrt(3)*cos(theta)  sin(theta)  -sin(theta) ; ...
                    -sqrt(3)*sin(theta)  cos(theta)  -cos(theta)];

Y_dq =PC_T*X_abc;
end

== matlab function LinearIntegralAntiWindup/SteerActuator/BLDCWRack/RackSubsystem/SteerMechanics ==
  data: dd input; dWs input; Ws input; Vx input; Ts output; m parameter; g parameter; t_f output; t_a output
function [Ts,t_f,t_a] = fcn(dd, dWs, Ws,Vx, m, g)

Fz = (m*g)/2; % N.  4 tires
J_s = 0.024; %kg
B_s = 0.00172; % Nm*s/deg
epsilon = 0.1;
Nl = 0.005;


t_f = -Fz * tanh(Ws/(epsilon)); % derivative of dd is equivalent 
    % to 1/Nm of the electrical angular speed
t_a = -Fz*Vx*sin(dd);


Ts = Nl*(J_s*dWs + B_s*Ws - t_a - t_f);

== matlab function LinearIntegralAntiWindup/SteerActuator/BLDC_AngleCtrl/BLDC abc model ==
  data: X input; f input; v input; dX output; Tl input; R parameter; L parameter; M parameter; J parameter; b parameter; P parameter; lambda parameter
function dX = fcn(X,f,v,Tl, R, L, M, J, b, P, lambda)
% X = [i_a; i_b; i_c; wm; theta_elec]
% f = [f1; f2; f3]  (0..1)
% v = [v1; v2; v3]  (example v = 12.*f)
% Tl = scalar torque load)
% lambda = ke = kt (V·s/rad = N·m/A)
% P = poles qty (pole pairs = P/2
%
% delivers dX = [di_a; di_b; di_c; dwm; dtheta_elec]

% sanity checks
if numel(f)~=3 || numel(v)~=3
    error('f and v must be vectors 3x1.');
end

% effective electric parameters
L_eff = L - M;
if L_eff <= 0
    error('L - M must be possitive. Check M.');
end


% states
i_a = X(1); i_b = X(2); i_c = X(3);
wm  = X(4); theta = X(5);


% electric equations (phase to phase)
di_a = ( v(1) - R*i_a - lambda * f(1) * wm ) / L_eff;
di_b = ( v(2) - R*i_b - lambda * f(2) * wm ) / L_eff;
di_c = ( v(3) - R*i_c - lambda * f(3) * wm ) / L_eff;

% Mechanic equations
T_elec = lambda*( f(1)*i_a + f(2)*i_b + f(3)*i_c ); % torque eléctrico
dwm = ( T_elec - b*wm - Tl ) / J;


% Electric angle
dtheta = (P/2) * wm;

dX = [di_a; di_b; di_c; dwm; dtheta];

end

== matlab function LinearIntegralAntiWindup/LateralController/HOSMC_AckermanSuperTwist/HOSMC_AckermanSuperTwis1 ==
  data: U output size=1; E input; Vx input; Mu1 input; C_af parameter; g parameter; C_ar parameter; lf parameter; lr parameter; Iz parameter; m parameter; dMu1 output
% ******************* Lateral dynamic controller *********************
%*********************************************************************
% Author: L.Arturo Torres-Romero
% Date: 22-10-2020
% This controller controlls the direction of a car, based in the dynamics
% described  in the next link and using the conventional sliding mode control 
% formulation with the procedure of converting to regular form: 
% https://www.researchgate.net/publication/340166902_LATERAL_VEHICLE_DYNAMICS_AND_CONTROLLERS_DESIGN
%******************* PARAMETERS DESCRIPTIONS **********************
%******************************************************************
% m: vehicle mass
% g: gravity
% C_af : Cornering  stiffness  of  front  wheels.
% C_ar : Cornering  stiffness  of  rear  wheels.
% lf : distance fron the center of gravity to the front wheel axis.
% lr : distance fron the center of gravity to the rear wheel axis.
% Iz : this is the momentum of inertia of the vehicle respect the z axis.
%******************************************************************
%******************* INPUTS DESCRIPTIONS **************************
%******************************************************************
% E:   (column vector)[e1;de1;e2;de2] states of the state space of 
%       the system that includes the errors as follows:
%      e1  : is the lateral position error respect the road.
%      de1 : derivative of e1.
%      e2  : is the yaw angle error with respect the road. 
%      de2 : derivarive of the e2.
% Vx: Logitudinal velocity.

%******************************************************************
% ******************* OUTPUTS DESCRIPTIONS ************************
%******************************************************************
% U: control coutput in radians. Angle of the frontal wheels respect to the
%    longitudinal axis
% isCtrl: when true means that the matrix Mc has full rank, and hence, the
%         system is controllable
%******************************************************************

function [U, dMu1] = SMC_AckermanSuperTwistingCtrl(E, Vx, Mu1,C_af, g, C_ar, lf, lr, Iz, m) % pd polos deseados
X = [0; 0; 0; 0];
X(1) = E(1);
X(2) = E(2);
X(3) = E(3);
X(4) = E(4);
%**************************************************
%******* Matrix A formulation *********************
A22 = -(2*C_af + 2*C_ar)/(m*Vx);
A23 = (2*C_af + 2*C_ar)/m;
A24 = (-2*C_af*lf + 2*C_ar*lr)/(m*Vx);
A42 = -(2*C_af*lf - 2*C_ar*lr)/(Iz*Vx);
A43 = (2*C_af*lf - 2*C_ar*lr)/Iz;
A44 = -(2*C_af*lf^2 + 2*C_ar*lr^2)/(Iz*Vx);

A = [0 1 0 0;0 A22 A23 A24;0 0 0 1;0 A42 A43 A44];
%**************************************************

%**************************************************
%******* Matrix B1 formulation ********************
B1_2 = 2*C_af/m;
B1_4 = 2*C_af*lf/Iz;

B1 = [0;B1_2;0;B1_4];
%***************************************************

%***************************************************
%******* Matrix B2 formulation *********************
B2_2 = -(2*C_af*lf - 2*C_ar*lr)/(m*Vx) - Vx;
B2_4 = -(2*C_af*lf^2 + 2*C_ar*lr^2)/(Iz*Vx);

B2 = [0;B2_2;0;B2_4];
%***************************************************


%***************************************************
%******* Matrix B3 formulation *********************
B3 = [0;g;0;0];
%***************************************************


%***************************************************
%******* Verification of controllability and output 
% calculation of the controller
%**************************************************
d_k = 0;
Mc = [B1 A*B1 A^2*B1 A^3*B1];
rankVal = rank(Mc);
    if rankVal < size(A,1)
        %disp('Not completely state controllable');
        isCtrl = 0;
        d_k = 0;
    else
        %disp('Completely state controllable');
        isCtrl = 1;
        % Pole placement
        %Pd =[-5-3i -5+3i -7 -10];
        Pd =[-5-5i -5+5i -7 -10];

        H = (A- Pd(1)*eye(4)) * (A- Pd(2)*eye(4)) * (A- Pd(3)*eye(4)) * (A- Pd(4)*eye(4));

        %ackerman formula
        K = [0 0 0 1]*Mc^-1*H;
        d_k = -K*X;  
    end

%*********** Controller parameters **************
k_smc = 100;   %10
sigma = 40;    %60
gamma1 = 1;
gamma2 = 1;
gamma = [0 gamma1 0 gamma2];

h_c = gamma*[0;3;0;3];
g_c = gamma*B1;
q = 0.3;

UM = abs(h_c/g_c)/q;

%***********************************************
e_c = gamma*[0; X(1);0;X(3)];
d_u = (-1/(gamma*B1))*(sigma*sqrt(abs(e_c))*sign(e_c) + Mu1);

if abs(Mu1) > UM 
   dMu1 = -Mu1;
else
   dMu1 = -k_smc*sign(e_c); 
end

ctrlVal = d_k + d_u;

U = real(ctrlVal);
